simulink model "delay_test"  (R2020a)
settings: Solver=VariableStepAuto  StartTime=0.0  StopTime=10.0  RelTol=1e-3
libraries: arduinolib x8, etargetslib x6
settings Model: Creator=imkis  LastModifiedBy=imkis

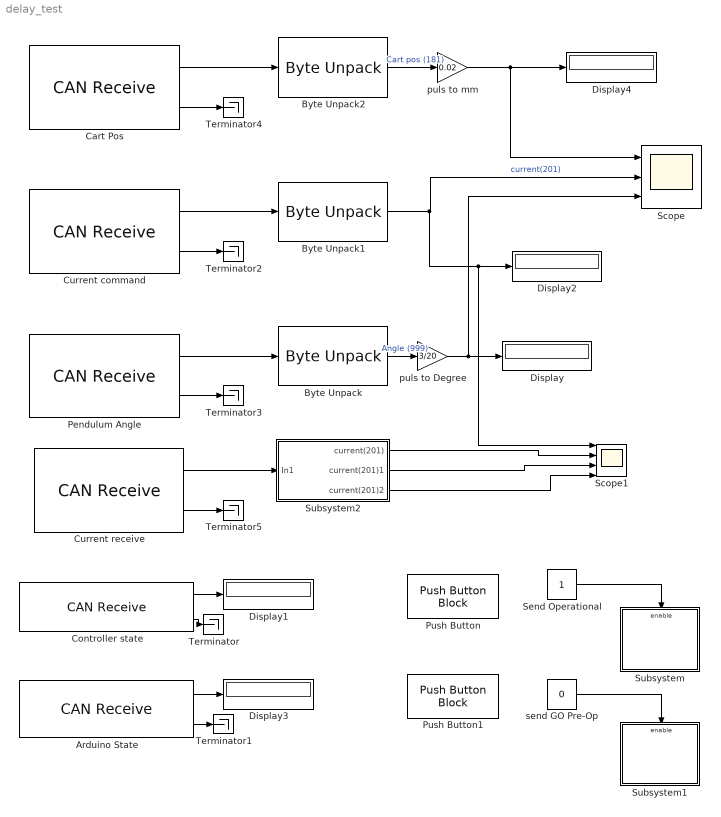
== system delay_test ==
  Arduino State : arduinolib/CAN Receive  outputDataType=Raw data  identifierType=Standard (11-bit identifier)  messageId=hex2dec('702')  msgLength=1  SampleTime=1  outputError=off  outputRemote=off
      settings: SourceProductBaseCode=ARDUINO
  Byte Unpack : etargetslib/Byte Unpack  dimensions={[1]}  datatypes={'int32'}  byteAlign=4
  Byte Unpack1 : etargetslib/Byte Unpack  dimensions={[1]}  datatypes={'int16'}  byteAlign=2
  Byte Unpack2 : etargetslib/Byte Unpack  dimensions={[1]}  datatypes={'int32'}  byteAlign=4
  Cart Pos : arduinolib/CAN Receive  outputDataType=Raw data  identifierType=Standard (11-bit identifier)  messageId=hex2dec('181')  msgLength=4  SampleTime=0.001  outputError=off  outputRemote=off
      settings: SourceProductBaseCode=ARDUINO
  Controller state : arduinolib/CAN Receive  outputDataType=Raw data  identifierType=Standard (11-bit identifier)  messageId=hex2dec('701')  msgLength=1  SampleTime=1  outputError=off  outputRemote=off
      settings: SourceProductBaseCode=ARDUINO
  Current command : arduinolib/CAN Receive  outputDataType=Raw data  identifierType=Standard (11-bit identifier)  messageId=hex2dec('201')  msgLength=2  SampleTime=0.001  outputError=off  outputRemote=off
      settings: SourceProductBaseCode=ARDUINO
  Current receive : arduinolib/CAN Receive  outputDataType=Raw data  identifierType=Standard (11-bit identifier)  messageId=hex2dec('281')  msgLength=6  SampleTime=0.001  outputError=off  outputRemote=off
      settings: SourceProductBaseCode=ARDUINO
  Display{,1..4} (5 alike) : Display
  Pendulum Angle : arduinolib/CAN Receive  outputDataType=Raw data  identifierType=Standard (11-bit identifier)  messageId=999  msgLength=4  SampleTime=0.001  outputError=off  outputRemote=off
      settings: SourceProductBaseCode=ARDUINO
  Push Button : PushButtonBlock  ButtonText=Go Operational
  Push Button1 : PushButtonBlock  ButtonText=GO Pre-Operational
  Scope : Scope  NumInputPorts=3
  Scope1 : Scope  NumInputPorts=4
  Send Operational : Constant
  Subsystem : Subsystem
  Subsystem1 : Subsystem
  Subsystem2 : Subsystem
  Terminator{,1..5} (6 alike) : Terminator
  puls to Degree : Gain  Gain=3/20
  puls to mm : Gain  Gain=0.02
  send GO Pre-Op : Constant  Value=0
  wires:
  puls to Degree/1 -> Display/1, Scope/3
  puls to mm/1 -> Display4/1, Scope/1
  Arduino State/2 -> Terminator1/1
  Pendulum Angle/2 -> Terminator3/1
  send GO Pre-Op/1 -> Subsystem1/Enable
  Byte Unpack2/1 -> puls to mm/1  "Cart pos (181)"
  Arduino State/1 -> Display3/1
  Controller state/2 -> Terminator/1
  Cart Pos/2 -> Terminator4/1
  Cart Pos/1 -> Byte Unpack2/1
  Byte Unpack1/1 -> Scope1/1, Display2/1, Scope/2  "current(201)"
  Controller state/1 -> Display1/1
  Current command/2 -> Terminator2/1
  Send Operational/1 -> Subsystem/Enable
  Current command/1 -> Byte Unpack1/1
  Byte Unpack/1 -> puls to Degree/1  "Angle (999)"
  Pendulum Angle/1 -> Byte Unpack/1
  Current receive/2 -> Terminator5/1
  Current receive/1 -> Subsystem2/1(In1)
  Subsystem2/1(current(201)) -> Scope1/2
  Subsystem2/2(current(201)1) -> Scope1/3
  Subsystem2/3(current(201)2) -> Scope1/4

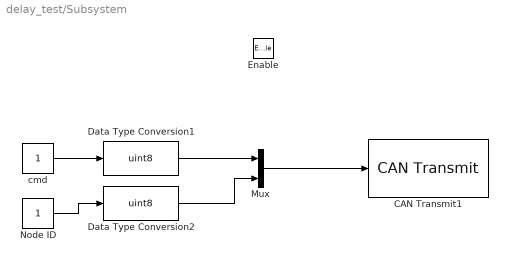
== system delay_test/Subsystem ==
  Enable : EnablePort
  CAN Transmit1 : arduinolib/CAN Transmit  inputDataType=Raw data  BlockingMode_=off  BlockTimeout_=1  outputStatus=off  identifierType=Standard (11-bit identifier)  messageId=0  msgLength=2  remoteFrame=off
      settings: SourceProductBaseCode=ARDUINO
  Data Type Conversion1 : DataTypeConversion  OutDataTypeStr=uint8
  Data Type Conversion2 : DataTypeConversion  OutDataTypeStr=uint8
  Mux : Mux  Inputs=2
  Node ID : Constant  SampleTime=2
  cmd : Constant  SampleTime=2
  wires:
  Data Type Conversion2/1 -> Mux/2
  Data Type Conversion1/1 -> Mux/1
  Mux/1 -> CAN Transmit1/1
  Node ID/1 -> Data Type Conversion2/1
  cmd/1 -> Data Type Conversion1/1

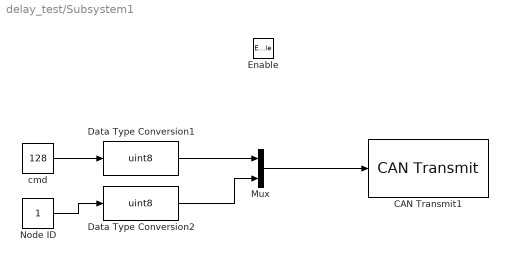
== system delay_test/Subsystem1 ==
  Enable : EnablePort
  CAN Transmit1 : arduinolib/CAN Transmit  inputDataType=Raw data  BlockingMode_=off  BlockTimeout_=1  outputStatus=off  identifierType=Standard (11-bit identifier)  messageId=0  msgLength=2  remoteFrame=off
      settings: SourceProductBaseCode=ARDUINO
  Data Type Conversion1 : DataTypeConversion  OutDataTypeStr=uint8
  Data Type Conversion2 : DataTypeConversion  OutDataTypeStr=uint8
  Mux : Mux  Inputs=2
  Node ID : Constant  SampleTime=1
  cmd : Constant  Value=128  SampleTime=1
  wires:
  Data Type Conversion2/1 -> Mux/2
  Data Type Conversion1/1 -> Mux/1
  Mux/1 -> CAN Transmit1/1
  Node ID/1 -> Data Type Conversion2/1
  cmd/1 -> Data Type Conversion1/1

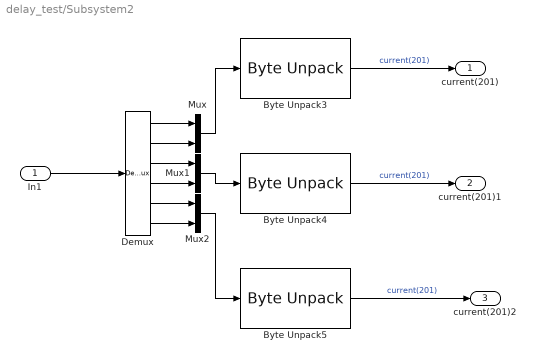
== system delay_test/Subsystem2 ==
  In1 : Inport
  Byte Unpack3 : etargetslib/Byte Unpack  dimensions={[1]}  datatypes={'int16'}  byteAlign=2
  Byte Unpack4 : etargetslib/Byte Unpack  dimensions={[1]}  datatypes={'int16'}  byteAlign=2
  Byte Unpack5 : etargetslib/Byte Unpack  dimensions={[1]}  datatypes={'int16'}  byteAlign=2
  Demux : Demux  Outputs=6
  Mux : Mux  Inputs=2
  Mux1 : Mux  Inputs=2
  Mux2 : Mux  Inputs=2
  current(201) : Outport
  current(201)1 : Outport  Port=2
  current(201)2 : Outport  Port=3
  wires:
  Demux/6 -> Mux2/2
  Demux/5 -> Mux2/1
  Demux/1 -> Mux/1
  Mux/1 -> Byte Unpack3/1
  Demux/2 -> Mux/2
  Mux1/1 -> Byte Unpack4/1
  Demux/4 -> Mux1/2
  Mux2/1 -> Byte Unpack5/1
  Demux/3 -> Mux1/1
  Byte Unpack3/1 -> current(201)/1  "current(201)"
  Byte Unpack5/1 -> current(201)2/1  "current(201)"
  Byte Unpack4/1 -> current(201)1/1  "current(201)"
  In1/1 -> Demux/1
